simulink model "FINAL"  (R2019a)
settings: Solver=VariableStepAuto  StartTime=0.0  StopTime=5  FixedStep=0.0001  RelTol=1e-3
PreLoadFcn:
  | initDuckWPT
InitFcn:
  | initDuckWPT
StartFcn:
  | initDuckWPT
values from neighbouring files (symbols this model uses):
  angleTolerance = 2    [initDuckWPT.m]
  eeTolerance = 0.01    [initDuckWPT.m]
  JointBounds1 = [-pi/2       pi ... (first row only)    [initDuckWPT.m]
  JointBounds2 = [-pi/3       pi/3 ... (first row only)    [initDuckWPT.m]
  rotM1 = roty(90)*rotx(90)    [initDuckWPT.m]
  trajectory = [0.4  0.4  0.4  0.4  0.4  0.4  0.4 ... (first row only)    [initDuckWPT.m]
undefined symbols (not defined in the file or in its folder): DiscIntNeverNeededParam, X, Y, Z
libraries: sm_lib x205, fl_lib x72, nesl_utility x43, fl_ps_legacy_lib x18, fuzblock x16, Contact_Forces_Lib x12
(part 1 of 7)
Description:
  | Two 7-DOF Robot Arm
  | Follow Trajectory Seperate 2 Arm, No Torque, No Grabbing
settings Model: PauseTimes=4  Creator=josea  LastModifiedBy=Duke Nguyen
settings DataIOCC: ReturnWorkspaceOutputs=off
settings DebuggingCC: PregeneratedLibrarySubsystemCodeDiagnostic=none  ArithmeticOperatorsInVariantConditions=warning
settings SFSimCC: SimUseLocalCustomCode=off
settings RTWCC: RTWUseLocalCustomCode=off
settings SimscapeCC: SimscapeLogType=all  SimscapeLogName=simlog_waypoint_tracking  SimscapeLogLimitData=off
settings ExplorerConfigSet: InternalSimMechanicsExplorerSettings="<ExplorerConfiguration><canonicalview>default</canonicalview><AnimationSetting><BasePlaybackSpeed>1.0</BasePlaybackSpeed><PlaybackSpeedFactor>1.0</PlaybackSpeedFactor></AnimationSetting><TilePanel><TileInfo><Tiles Columns=\"2\" Count=\"3\" Rows=\"2\"><Column Weight=\"0.523\"/><Column Weight=\"0.477\"/><Row Weight=\"0.4994\"/><Row Weight=\"0.5006\"/><Tile Height=\"2\" Width=\"1\" X=\"0\" Y=\"0\"/><Tile Height=\"1\" Width=\"1\" X=\"1\" Y=\"0\"/><Tile Height=\"1\" Width=\"1\" X=\"1\" Y=\"1\"/></Tiles></TileInfo><SceneInfo><SceneViewer><BGColor><R>0.800000011920928955</R><G>0.800000011920928955</G><B>0.800000011920928955</B></BGColor><Camera><DoPerspective>off</DoPerspective><Position><X>1.19928295196616075</X><Y>-0.370963369649593755</Y><Z>0.192902442559522713</Z></Position><Center><X>0.466827313465554616</X><Y>0.0298302780043228633</Y><Z>-0.357436716168019419</Z></Center><Up><X>-0.458278077763030423</X><Y>0.307545069196018872</Y><Z>0.833904811027636583</Z></Up><ViewLimDist>1</ViewLimDist><YLim>0.756041493589077906</YLim><XLim>0.742600755925272082</XLim></Camera></SceneViewer><SceneViewer><BGColor><R>0.800000011920928955</R><G>0.800000011920928955</G><B>0.800000011920928955</B></BGColor><Camera><DoPerspective>off</DoPerspective><Position><X>1.51688776390650482</X><Y>-1.12635047955222944e-08</Y><Z>-0.248862136929848043</Z></Position><Center><X>0.453640252731354554</X><Y>-1.12635047955222944e-08</Y><Z>-0.248862136929848043</Z></Center><Up><X>-0</X><Y>0</Y><Z>1</Z></Up><ViewLimDist>1</ViewLimDist><YLim>0.361672012805938747</YLim><XLim>0.655073353531655411</XLim></Camera></SceneViewer><SceneViewer><BGColor><R>0.800000011920928955</R><G>0.800000011920928955</G><B>0.800000011920928955</B></BGColor><Camera><DoPerspective>off</DoPerspective><Position><X>0.45769736697222041</X><Y>-1.00000001614500644</Y><Z>-0.253455854452269813</Z></Position><Center><X>0.45769736697222041</X><Y>-1.61450063873580518e-08</Y><Z>-0.253455854452269813</Z></Center><Up><X>0</X><Y>-0</Y><Z>1</Z></Up><ViewLimDist>1</ViewLimDist><YLim>0.356940470933914178</YLim><XLim>0.645053855544248544</XLim></Camera></SceneViewer></SceneInfo></TilePanel><MechEditorPanel><Cameras/><GfxPanelCameraMap/><VideoCreator><PlaybackSpeedRatio>1.0</PlaybackSpeedRatio><FrameRate>30</FrameRate><VideoFormat>Motion JPEG AVI</VideoFormat><FrameSize>auto</FrameSize></VideoCreator></MechEditorPanel></ExplorerConfiguration>"

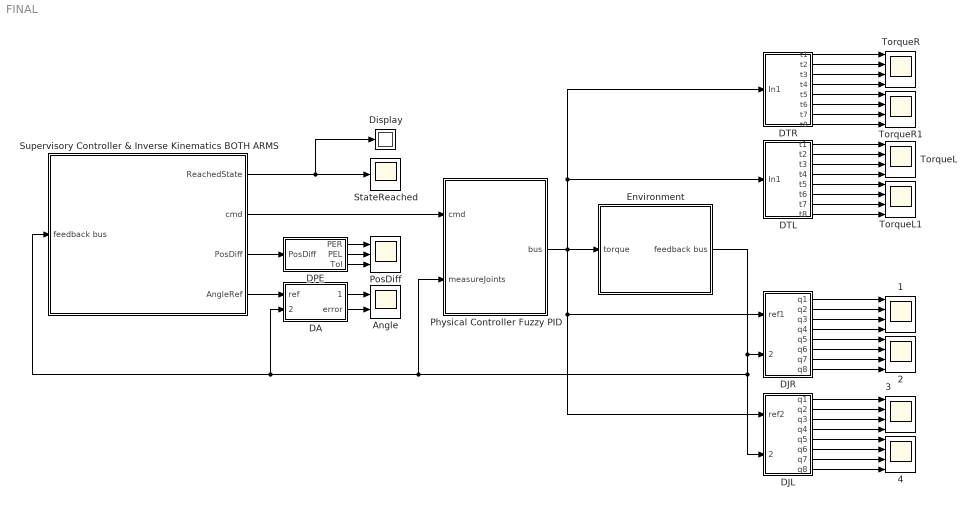
== system FINAL ==
  {1..4} (4 alike) : Scope  NumInputPorts=4
  Angle : Scope  NumInputPorts=2
  DA : Subsystem
  DJL : Subsystem
  DJR : Subsystem
  DPE : Subsystem
  DTL : Subsystem
  DTR : Subsystem
  Display : Display
  Environment : Subsystem
      mask Display: image('envi.png');
  Physical Controller Fuzzy PID : Subsystem
  PosDiff : Scope  NumInputPorts=3
  StateReached : Scope
  Supervisory Controller & Inverse Kinematics BOTH ARMS : Subsystem
  TorqueL : Scope  NumInputPorts=4
  TorqueL1 : Scope  NumInputPorts=4
  TorqueR : Scope  NumInputPorts=4
  TorqueR1 : Scope  NumInputPorts=4
  wires:
  Environment/1(feedback bus) -> Physical Controller Fuzzy PID/2(measureJoints), Supervisory Controller & Inverse Kinematics BOTH ARMS/1(feedback bus), DA/2(angle), DJL/2(meas), DJR/2(meas)
  Physical Controller Fuzzy PID/1(bus) -> DJL/1(ref2), DJR/1(ref1), Environment/1(torque), DTR/1(In1), DTL/1(In1)
  DA/1(tracking) -> Angle/1
  DA/2(error) -> Angle/2
  Supervisory Controller & Inverse Kinematics BOTH ARMS/1(ReachedState) -> Display/1, StateReached/1
  Supervisory Controller & Inverse Kinematics BOTH ARMS/3(PosDiff) -> DPE/1(PosDiff)
  DPE/1(PER) -> PosDiff/1
  DPE/2(PEL) -> PosDiff/2
  DPE/3(Tol) -> PosDiff/3
  Supervisory Controller & Inverse Kinematics BOTH ARMS/2(cmd) -> Physical Controller Fuzzy PID/1(cmd)
  Supervisory Controller & Inverse Kinematics BOTH ARMS/4(AngleRef) -> DA/1(ref)
  DTR/1(t1) -> TorqueR/1
  DTR/2(t2) -> TorqueR/2
  DTR/3(t3) -> TorqueR/3
  DTR/4(t4) -> TorqueR/4
  DTR/5(t5) -> TorqueR1/1
  DTR/6(t6) -> TorqueR1/2
  DTR/7(t7) -> TorqueR1/3
  DTR/8(t8) -> TorqueR1/4
  DTL/1(t1) -> TorqueL/1
  DTL/2(t2) -> TorqueL/2
  DTL/3(t3) -> TorqueL/3
  DTL/4(t4) -> TorqueL/4
  DTL/5(t5) -> TorqueL1/1
  DTL/6(t6) -> TorqueL1/2
  DTL/7(t7) -> TorqueL1/3
  DTL/8(t8) -> TorqueL1/4
  DJR/1(q1) -> 1/1
  DJR/2(q2) -> 1/2
  DJR/3(q3) -> 1/3
  DJR/4(q4) -> 1/4
  DJR/5(q5) -> 2/1
  DJR/6(q6) -> 2/2
  DJR/7(q7) -> 2/3
  DJR/8(q8) -> 2/4
  DJL/1(q1) -> 3/1
  DJL/2(q2) -> 3/2
  DJL/3(q3) -> 3/3
  DJL/4(q4) -> 3/4
  DJL/5(q5) -> 4/1
  DJL/6(q6) -> 4/2
  DJL/7(q7) -> 4/3
  DJL/8(q8) -> 4/4

== system FINAL/DA ==
  ref : Inport
  angle : Inport  Port=2
  Abs : Abs
  Bus Selector2 : BusSelector  OutputSignals=ObjectAngle
  Constant : Constant  Value=angleTolerance
  Mux : Mux  Inputs=2
  Mux1 : Mux  Inputs=2
  Subtract : Sum  Inputs=+-
  tracking : Outport
  error : Outport  Port=2
  wires:
  ref/1 -> Subtract/1, Mux/1
  Mux/1 -> tracking/1
  angle/1 -> Bus Selector2/1
  Bus Selector2/1 -> Subtract/2, Mux/2  "<ObjectAngle>"
  Subtract/1 -> Abs/1
  Constant/1 -> Mux1/2
  Mux1/1 -> error/1
  Abs/1 -> Mux1/1

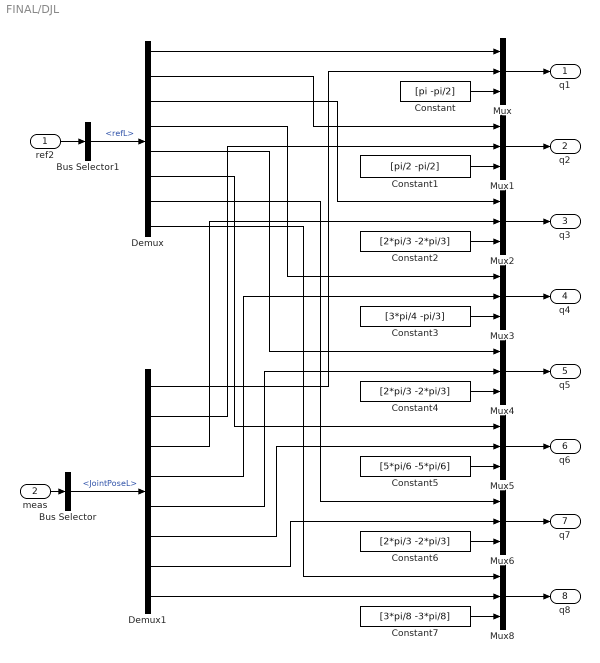
== system FINAL/DJL ==
  ref2 : Inport
  meas : Inport  Port=2
  Bus Selector : BusSelector  OutputSignals=JointPoseL
  Bus Selector1 : BusSelector  OutputSignals=refL
  Constant : Constant  Value=[pi -pi/2]
  Constant1 : Constant  Value=[pi/2 -pi/2]
  Constant2 : Constant  Value=[2*pi/3 -2*pi/3]
  Constant3 : Constant  Value=[3*pi/4 -pi/3]
  Constant4 : Constant  Value=[2*pi/3 -2*pi/3]
  Constant5 : Constant  Value=[5*pi/6 -5*pi/6]
  Constant6 : Constant  Value=[2*pi/3 -2*pi/3]
  Constant7 : Constant  Value=[3*pi/8 -3*pi/8]
  Demux : Demux  Outputs=8
  Demux1 : Demux  Outputs=8
  Mux{,1..6,8} (8 alike) : Mux  Inputs=3
  q1 : Outport
  q2 : Outport  Port=2
  q3 : Outport  Port=3
  q4 : Outport  Port=4
  q5 : Outport  Port=5
  q6 : Outport  Port=6
  q7 : Outport  Port=7
  q8 : Outport  Port=8
  wires:
  Bus Selector/1 -> Demux1/1  "<JointPoseL>"
  meas/1 -> Bus Selector/1
  Constant7/1 -> Mux8/3
  Demux/1 -> Mux/1
  Demux/2 -> Mux1/1
  Demux/3 -> Mux2/1
  Demux/4 -> Mux3/1
  Demux/5 -> Mux4/1
  Demux/6 -> Mux5/1
  Demux/7 -> Mux6/1
  Demux/8 -> Mux8/1
  Demux1/1 -> Mux/2
  Demux1/2 -> Mux1/2
  Demux1/3 -> Mux2/2
  Demux1/4 -> Mux3/2
  Demux1/5 -> Mux4/2
  Demux1/6 -> Mux5/2
  Demux1/7 -> Mux6/2
  Demux1/8 -> Mux8/2
  Constant/1 -> Mux/3
  Constant1/1 -> Mux1/3
  Constant2/1 -> Mux2/3
  Constant3/1 -> Mux3/3
  Constant4/1 -> Mux4/3
  Constant6/1 -> Mux6/3
  Constant5/1 -> Mux5/3
  Mux/1 -> q1/1
  Mux1/1 -> q2/1
  Mux2/1 -> q3/1
  Mux3/1 -> q4/1
  Mux5/1 -> q6/1
  Mux6/1 -> q7/1
  Mux8/1 -> q8/1
  Mux4/1 -> q5/1
  ref2/1 -> Bus Selector1/1
  Bus Selector1/1 -> Demux/1  "<refL>"

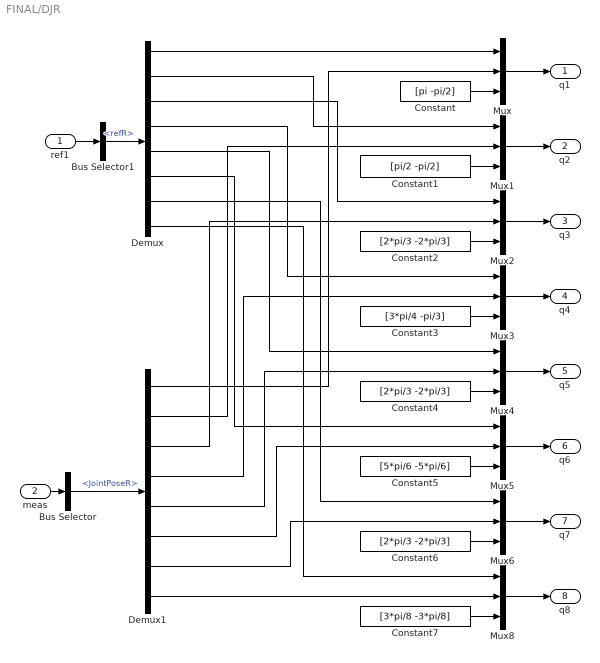
== system FINAL/DJR ==
  ref1 : Inport
  meas : Inport  Port=2
  Bus Selector : BusSelector  OutputSignals=JointPoseR
  Bus Selector1 : BusSelector  OutputSignals=refR
  Constant : Constant  Value=[pi -pi/2]
  Constant1 : Constant  Value=[pi/2 -pi/2]
  Constant2 : Constant  Value=[2*pi/3 -2*pi/3]
  Constant3 : Constant  Value=[3*pi/4 -pi/3]
  Constant4 : Constant  Value=[2*pi/3 -2*pi/3]
  Constant5 : Constant  Value=[5*pi/6 -5*pi/6]
  Constant6 : Constant  Value=[2*pi/3 -2*pi/3]
  Constant7 : Constant  Value=[3*pi/8 -3*pi/8]
  Demux : Demux  Outputs=8
  Demux1 : Demux  Outputs=8
  Mux{,1..6,8} (8 alike) : Mux  Inputs=3
  q1 : Outport
  q2 : Outport  Port=2
  q3 : Outport  Port=3
  q4 : Outport  Port=4
  q5 : Outport  Port=5
  q6 : Outport  Port=6
  q7 : Outport  Port=7
  q8 : Outport  Port=8
  wires:
  Mux4/1 -> q5/1
  Mux8/1 -> q8/1
  Mux6/1 -> q7/1
  Mux5/1 -> q6/1
  Mux3/1 -> q4/1
  Mux2/1 -> q3/1
  Mux1/1 -> q2/1
  Mux/1 -> q1/1
  Constant5/1 -> Mux5/3
  Constant6/1 -> Mux6/3
  Constant4/1 -> Mux4/3
  Constant3/1 -> Mux3/3
  Constant2/1 -> Mux2/3
  Constant1/1 -> Mux1/3
  Constant/1 -> Mux/3
  Demux1/8 -> Mux8/2
  Demux1/7 -> Mux6/2
  Demux1/6 -> Mux5/2
  Demux1/5 -> Mux4/2
  Demux1/4 -> Mux3/2
  Demux1/3 -> Mux2/2
  Demux1/2 -> Mux1/2
  Demux1/1 -> Mux/2
  Demux/8 -> Mux8/1
  Demux/7 -> Mux6/1
  Demux/6 -> Mux5/1
  Demux/5 -> Mux4/1
  Demux/4 -> Mux3/1
  Demux/3 -> Mux2/1
  Demux/2 -> Mux1/1
  Demux/1 -> Mux/1
  Constant7/1 -> Mux8/3
  meas/1 -> Bus Selector/1
  Bus Selector/1 -> Demux1/1  "<JointPoseR>"
  ref1/1 -> Bus Selector1/1
  Bus Selector1/1 -> Demux/1  "<refR>"

== system FINAL/DPE ==
  PosDiff : Inport
  Bus Selector : BusSelector  OutputSignals=PosDiffR,PosDiffL
  Constant6 : Constant  Value=eeTolerance
  Vector Length1 : Subsystem
  Vector Length2 : Subsystem
  PER : Outport
  PEL : Outport  Port=2
  Tol : Outport  Port=3
  wires:
  Bus Selector/1 -> Vector Length1/1(v)  "<PosDiffR>"
  PosDiff/1 -> Bus Selector/1
  Bus Selector/2 -> Vector Length2/1(v)  "<PosDiffL>"
  Vector Length1/1(r) -> PER/1
  Vector Length2/1(r) -> PEL/1
  Constant6/1 -> Tol/1

== system FINAL/DTL ==
  In1 : Inport
  Bus Selector3 : BusSelector  OutputSignals=torqueL
  Demux : Demux  Outputs=8
  t1 : Outport
  t2 : Outport  Port=2
  t3 : Outport  Port=3
  t4 : Outport  Port=4
  t5 : Outport  Port=5
  t6 : Outport  Port=6
  t7 : Outport  Port=7
  t8 : Outport  Port=8
  wires:
  In1/1 -> Bus Selector3/1
  Demux/4 -> t4/1
  Demux/1 -> t1/1
  Demux/7 -> t7/1
  Demux/3 -> t3/1
  Bus Selector3/1 -> Demux/1  "<torqueL>"
  Demux/2 -> t2/1
  Demux/5 -> t5/1
  Demux/8 -> t8/1
  Demux/6 -> t6/1

== system FINAL/DTR ==
  In1 : Inport
  Bus Selector2 : BusSelector  OutputSignals=torqueR
  Demux : Demux  Outputs=8
  t1 : Outport
  t2 : Outport  Port=2
  t3 : Outport  Port=3
  t4 : Outport  Port=4
  t5 : Outport  Port=5
  t6 : Outport  Port=6
  t7 : Outport  Port=7
  t8 : Outport  Port=8
  wires:
  Demux/6 -> t6/1
  Demux/4 -> t4/1
  Demux/2 -> t2/1
  Demux/5 -> t5/1
  In1/1 -> Bus Selector2/1
  Demux/7 -> t7/1
  Bus Selector2/1 -> Demux/1  "<torqueR>"
  Demux/3 -> t3/1
  Demux/8 -> t8/1
  Demux/1 -> t1/1

== system FINAL/Environment ==
  torque : Inport
  " " : Subsystem
  Bus Creator : BusCreator  Inputs=8
  Bus Selector : BusSelector  OutputSignals=torqueR,torqueL
  EE Position to World Base : Subsystem
  Rate Transition{,2,4..5} (4 alike) : RateTransition
  Robot : Subsystem  mask{damping_coefficient=2, damping_coefficient_gripper=0.14}
      mask prompts: damping_coefficient "Damping Coefficient"; damping_coefficient_gripper "Damping Coefficient Gripper"
  World : Subsystem  mask{ball_radius=3.5, contact_gripper_planeLength_x=0.05, contact_gripper_planeLength_y=0.7, contact_gripper_planeDepth=0.05, contact_gripper_stiffness=1000, contact_gripper_damping=70, contact_gripper_kFrictionCoeff=0.5, contact_gripper_sFrictionCoeff=0.72}
      mask prompts: ball_radius "Ball Radius"; contact_gripper_planeLength_x "Contact Gripper Plane Length X"; contact_gripper_planeLength_y "Contact Gripper Plane Length Y"; contact_gripper_planeDepth "Contact Gripper Plane Depth"; contact_gripper_stiffness "Contact Gripper Stiffness"; contact_gripper_damping "Contact Gripper Damping"; contact_gripper_kFrictionCoeff "Contact Gripper Kinematic Friction"; contact_gripper_sFrictionCoeff "Contact Gripper Static Friction"
  trajectoryL : ToWorkspace  VariableName=simout1  SaveFormat=Timeseries  SampleTime=-1
  trajectoryR : ToWorkspace  VariableName=simout  SaveFormat=Timeseries  SampleTime=-1
  feedback bus : Outport
  wires:
  Rate Transition/1 -> Bus Creator/1  "JointPoseR"
  Rate Transition2/1 -> Bus Creator/2  "JointPoseL"
  EE Position to World Base/1(EE1 Pos) -> Rate Transition4/1
  EE Position to World Base/2(EE2 Pos) -> Rate Transition5/1
  Rate Transition4/1 -> Bus Creator/3, trajectoryR/1  "EERPos"
  Rate Transition5/1 -> trajectoryL/1, Bus Creator/4  "EELPose"
  Robot/1(SensorData1) -> Rate Transition/1
  Robot/2(SensorData2) -> Rate Transition2/1
  World/1(ObjectPosition) -> Bus Creator/5  "Object Position"
  World/3(GripperForce2) -> Bus Creator/7  "GripForceL"
  World/2(GripperForce1) -> Bus Creator/6  "GripForceR"
  Bus Creator/1 -> feedback bus/1
  World/4(ObjectAngle) -> Bus Creator/8  "ObjectAngle"
  torque/1 -> Bus Selector/1
  Bus Selector/1 -> Robot/1(commandsRight)  "<torqueR>"
  Bus Selector/2 -> Robot/2(commandsLeft)  "<torqueL>"
  connections:
  Robot/LConn2 -- EE Position to World Base/LConn1
  Robot/LConn3 -- EE Position to World Base/LConn2
  " "/RConn1 -- World/LConn1 -- EE Position to World Base/LConn3 -- Robot/LConn1
  Robot/RConn1 -- World/RConn1
  Robot/RConn2 -- World/RConn3
  Robot/RConn3 -- World/RConn2
  World/RConn4 -- Robot/RConn4

== system FINAL/Physical Controller Fuzzy PID ==
  cmd : Inport
  measureJoints : Inport  Port=2
  Bus Creator : BusCreator  Inputs=4
  Bus Selector : BusSelector  OutputSignals=JointPoseR,JointPoseL
  Bus Selector1 : BusSelector  OutputSignals=DesiredJointStatesR,GripCommand,DesiredJointStatesL
  Fuzzy PID Tuning1 : Subsystem
  Fuzzy PID Tuning2 : Subsystem
  Grip Transition : Subsystem
  Mux1 : Mux  Inputs=2
  Mux2 : Mux  Inputs=2
  bus : Outport
  wires:
  Fuzzy PID Tuning1/1(Out1) -> Bus Creator/2  "torqueR"
  Fuzzy PID Tuning2/1(Out1) -> Bus Creator/3  "torqueL"
  Bus Selector1/2 -> Grip Transition/1(GripCmd)  "<GripCommand>"
  Bus Selector1/3 -> Mux1/1  "<DesiredJointStatesL>"
  Bus Selector/2 -> Fuzzy PID Tuning2/2(In2)  "<JointPoseL>"
  Grip Transition/1(GripRef) -> Mux2/2, Mux1/2
  Mux2/1 -> Fuzzy PID Tuning1/1(In1), Bus Creator/1  "refR"
  Bus Selector1/1 -> Mux2/1  "<DesiredJointStatesR>"
  Bus Creator/1 -> bus/1
  Bus Selector/1 -> Fuzzy PID Tuning1/2(In2)  "<JointPoseR>"
  Mux1/1 -> Fuzzy PID Tuning2/1(In1), Bus Creator/4  "refL"
  cmd/1 -> Bus Selector1/1
  measureJoints/1 -> Bus Selector/1

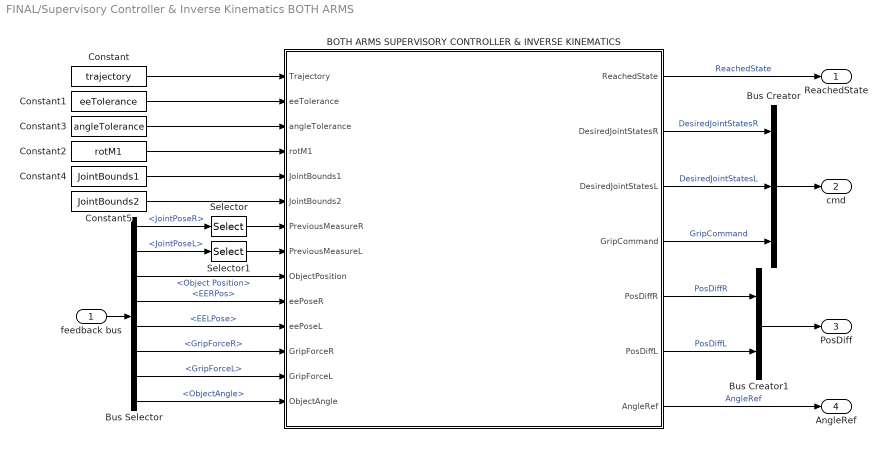
== system FINAL/Supervisory Controller & Inverse Kinematics BOTH ARMS ==
  feedback bus : Inport
  BOTH ARMS SUPERVISORY CONTROLLER & INVERSE KINEMATICS : Stateflow chart  TreatAsAtomicUnit=on
  Bus Creator : BusCreator  Inputs=3
  Bus Creator1 : BusCreator  Inputs=2
  Bus Selector : BusSelector  OutputSignals=JointPoseR,JointPoseL,Object Position,EERPos,EELPose,GripForceR,GripForceL,ObjectAngle
  Constant : Constant  Value=trajectory
  Constant1 : Constant  Value=eeTolerance
  Constant2 : Constant  Value=rotM1
  Constant3 : Constant  Value=angleTolerance
  Constant4 : Constant  Value=JointBounds1
  Constant5 : Constant  Value=JointBounds2
  Selector : Selector  InputPortWidth=8  IndexOptions=Index vector (dialog)  Indices=[1:7]  OutputSizes=1
  Selector1 : Selector  InputPortWidth=8  IndexOptions=Index vector (dialog)  Indices=[1:7]  OutputSizes=1
  ReachedState : Outport
  cmd : Outport  Port=2
  PosDiff : Outport  Port=3
  AngleRef : Outport  Port=4
  wires:
  Selector/1 -> BOTH ARMS SUPERVISORY CONTROLLER & INVERSE KINEMATICS/7(PreviousMeasureR)
  Constant2/1 -> BOTH ARMS SUPERVISORY CONTROLLER & INVERSE KINEMATICS/4(rotM1)
  Bus Selector/6 -> BOTH ARMS SUPERVISORY CONTROLLER & INVERSE KINEMATICS/12(GripForceR)  "<GripForceR>"
  Constant5/1 -> BOTH ARMS SUPERVISORY CONTROLLER & INVERSE KINEMATICS/6(JointBounds2)
  feedback bus/1 -> Bus Selector/1
  Constant1/1 -> BOTH ARMS SUPERVISORY CONTROLLER & INVERSE KINEMATICS/2(eeTolerance)
  Constant/1 -> BOTH ARMS SUPERVISORY CONTROLLER & INVERSE KINEMATICS/1(Trajectory)
  Constant4/1 -> BOTH ARMS SUPERVISORY CONTROLLER & INVERSE KINEMATICS/5(JointBounds1)
  Selector1/1 -> BOTH ARMS SUPERVISORY CONTROLLER & INVERSE KINEMATICS/8(PreviousMeasureL)
  Bus Selector/2 -> Selector1/1  "<JointPoseL>"
  Bus Selector/7 -> BOTH ARMS SUPERVISORY CONTROLLER & INVERSE KINEMATICS/13(GripForceL)  "<GripForceL>"
  Bus Selector/5 -> BOTH ARMS SUPERVISORY CONTROLLER & INVERSE KINEMATICS/11(eePoseL)  "<EELPose>"
  Bus Selector/1 -> Selector/1  "<JointPoseR>"
  Bus Selector/3 -> BOTH ARMS SUPERVISORY CONTROLLER & INVERSE KINEMATICS/9(ObjectPosition)  "<Object Position>"
  Bus Selector/8 -> BOTH ARMS SUPERVISORY CONTROLLER & INVERSE KINEMATICS/14(ObjectAngle)  "<ObjectAngle>"
  Bus Selector/4 -> BOTH ARMS SUPERVISORY CONTROLLER & INVERSE KINEMATICS/10(eePoseR)  "<EERPos>"
  BOTH ARMS SUPERVISORY CONTROLLER & INVERSE KINEMATICS/2(DesiredJointStatesR) -> Bus Creator/1  "DesiredJointStatesR"
  BOTH ARMS SUPERVISORY CONTROLLER & INVERSE KINEMATICS/3(DesiredJointStatesL) -> Bus Creator/2  "DesiredJointStatesL"
  BOTH ARMS SUPERVISORY CONTROLLER & INVERSE KINEMATICS/4(GripCommand) -> Bus Creator/3  "GripCommand"
  BOTH ARMS SUPERVISORY CONTROLLER & INVERSE KINEMATICS/1(ReachedState) -> ReachedState/1  "ReachedState"
  Bus Creator/1 -> cmd/1
  BOTH ARMS SUPERVISORY CONTROLLER & INVERSE KINEMATICS/5(PosDiffR) -> Bus Creator1/1  "PosDiffR"
  BOTH ARMS SUPERVISORY CONTROLLER & INVERSE KINEMATICS/6(PosDiffL) -> Bus Creator1/2  "PosDiffL"
  Bus Creator1/1 -> PosDiff/1
  BOTH ARMS SUPERVISORY CONTROLLER & INVERSE KINEMATICS/7(AngleRef) -> AngleRef/1  "AngleRef"
  Constant3/1 -> BOTH ARMS SUPERVISORY CONTROLLER & INVERSE KINEMATICS/3(angleTolerance)

== system FINAL/DPE/Vector Length1 ==
  v : Inport
  Demux : Demux  Outputs=3
  Sqrt : Sqrt  SaturateOnIntegerOverflow=on
  Square : Math  Operator=square  SaturateOnIntegerOverflow=on
  Square1 : Math  Operator=square  SaturateOnIntegerOverflow=on
  Square2 : Math  Operator=square  SaturateOnIntegerOverflow=on
  Sum : Sum  Inputs=+++
  r : Outport
  wires:
  Square1/1 -> Sum/2
  Sqrt/1 -> r/1
  Demux/3 -> Square2/1
  Sum/1 -> Sqrt/1
  v/1 -> Demux/1
  Demux/2 -> Square1/1
  Demux/1 -> Square/1
  Square2/1 -> Sum/3
  Square/1 -> Sum/1

== system FINAL/DPE/Vector Length2 ==
  v : Inport
  Demux : Demux  Outputs=3
  Sqrt : Sqrt  SaturateOnIntegerOverflow=on
  Square : Math  Operator=square  SaturateOnIntegerOverflow=on
  Square1 : Math  Operator=square  SaturateOnIntegerOverflow=on
  Square2 : Math  Operator=square  SaturateOnIntegerOverflow=on
  Sum : Sum  Inputs=+++
  r : Outport
  wires:
  Square/1 -> Sum/1
  Square2/1 -> Sum/3
  Demux/1 -> Square/1
  Demux/2 -> Square1/1
  v/1 -> Demux/1
  Sum/1 -> Sqrt/1
  Demux/3 -> Square2/1
  Sqrt/1 -> r/1
  Square1/1 -> Sum/2

== system FINAL/Environment/  ==
  MechanismConfiguration : sm_lib/Utilities/Mechanism Configuration  UniformGravity=Constant  GravityVector=[0 0 -9.80665]  GravityUnits=m/s^2  LinearizationDelta=0.001
  Solver Configuration : nesl_utility/Solver Configuration  PhysicalDomain=network_engine_domain  SubClassName=solver  LeftPortType=input  RightPortType=generic  Tones=[]  Harmonics=[]  SimulateNoise=off  Profile=off  UseLocalSampling=off  EnableSwitchedLinearOptims=on  FrequencyDomain=off  UseCCode=off  RelTol=0.001  AbsTol=1e-06  MinStep=1e-09  ToWorkspace=off  RevertToSquareIcSolve=off  NumHomotopyIterations=100  PhasorMode=off  PhasorModeNumHarmonics=1  DoDC=off  ResidualTolerance=1e-09  UseLocalSolver=off  LocalSolverChoice=NE_BACKWARD_EULER_ADVANCER  LocalSolverSampleTime=0.001  DoFixedCost=off  MaxNonlinIter=3  MaxModeIter=2  LinearAlgebra=Sparse  EquationFormulation=NE_TIME_EF  DelaysMemoryBudget=1024  AutomaticFiltering=on  FilteringTimeConstant=0.001  PartitionStorageMethod=AS_NEEDED  PartitionMemoryBudget=1024  PartitionMethod=FAST
  World1 : sm_lib/Frames and Transforms/World Frame
  WC : PMIOPort  Side=Right
  connections:
  World1/RConn1 -- WC/RConn1 -- Solver Configuration/RConn1 -- MechanismConfiguration/RConn1

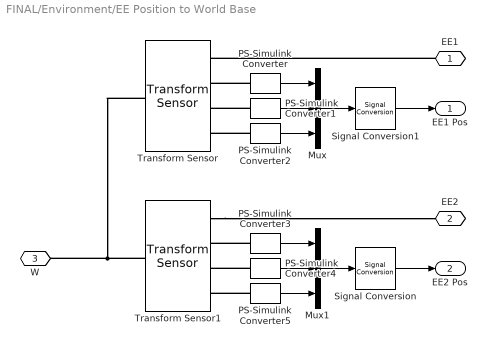
== system FINAL/Environment/EE Position to World Base ==
  Mux : Mux  Inputs=3
  Mux1 : Mux  Inputs=3
  PS-Simulink Converter{,1..5} (6 alike) : nesl_utility/PS-Simulink Converter  PhysicalDomain=network_engine_domain  SubClassName=ps_output  LeftPortType=input  RightPortType=output  PseudoPeriodic=off  Frequencies=[]  Unit=1  AffineConversion=off
  Signal Conversion : SignalConversion  OverrideOpt=off
  Signal Conversion1 : SignalConversion  OverrideOpt=off
  Transform Sensor : sm_lib/Frames and Transforms/Transform Sensor  MeasurementFrame=World  SenseAngle=off  SenseAxis=off  SenseAngle1=off  SenseAngle2=off  SenseAngle3=off  SenseQ=off  SenseR=off  SenseOmegaX=off  SenseOmegaY=off  SenseOmegaZ=off  SenseOmega1=off  SenseOmega2=off  SenseOmega3=off  SenseQDot=off  SenseRDot=off  SenseAlphaX=off  SenseAlphaY=off  SenseAlphaZ=off  SenseAlpha1=off  SenseAlpha2=off  SenseAlpha3=off  SenseQDDot=off  SenseRDDot=off  SenseX=on  SenseY=on  SenseZ=on  SenseRad=off  SenseAzim=off  SenseDist=off  SenseInc=off  SenseXDot=off  SenseYDot=off  SenseZDot=off  SenseRadDot=off  SenseAzimDot=off  SenseDistDot=off  SenseIncDot=off  SenseXDDot=off  SenseYDDot=off  SenseZDDot=off  SenseRadDDot=off  SenseAzimDDot=off  SenseDistDDot=off  SenseIncDDot=off
  Transform Sensor1 : sm_lib/Frames and Transforms/Transform Sensor  MeasurementFrame=World  SenseAngle=off  SenseAxis=off  SenseAngle1=off  SenseAngle2=off  SenseAngle3=off  SenseQ=off  SenseR=off  SenseOmegaX=off  SenseOmegaY=off  SenseOmegaZ=off  SenseOmega1=off  SenseOmega2=off  SenseOmega3=off  SenseQDot=off  SenseRDot=off  SenseAlphaX=off  SenseAlphaY=off  SenseAlphaZ=off  SenseAlpha1=off  SenseAlpha2=off  SenseAlpha3=off  SenseQDDot=off  SenseRDDot=off  SenseX=on  SenseY=on  SenseZ=on  SenseRad=off  SenseAzim=off  SenseDist=off  SenseInc=off  SenseXDot=off  SenseYDot=off  SenseZDot=off  SenseRadDot=off  SenseAzimDot=off  SenseDistDot=off  SenseIncDot=off  SenseXDDot=off  SenseYDDot=off  SenseZDDot=off  SenseRadDDot=off  SenseAzimDDot=off  SenseDistDDot=off  SenseIncDDot=off
  EE1 : PMIOPort  Side=Left
  EE2 : PMIOPort  Port=2  Side=Left
  W : PMIOPort  Port=3  Side=Left
  EE1 Pos : Outport
  EE2 Pos : Outport  Port=2
  wires:
  PS-Simulink Converter1/1 -> Mux/2
  PS-Simulink Converter3/1 -> Mux1/1
  PS-Simulink Converter/1 -> Mux/1
  PS-Simulink Converter2/1 -> Mux/3
  PS-Simulink Converter4/1 -> Mux1/2
  PS-Simulink Converter5/1 -> Mux1/3
  Mux/1 -> Signal Conversion1/1
  Mux1/1 -> Signal Conversion/1
  Signal Conversion/1 -> EE2 Pos/1
  Signal Conversion1/1 -> EE1 Pos/1
  connections:
  PS-Simulink Converter5/LConn1 -- Transform Sensor1/RConn4
  PS-Simulink Converter3/LConn1 -- Transform Sensor1/RConn2
  Transform Sensor1/LConn1 -- Transform Sensor/LConn1 -- W/RConn1
  EE1/RConn1 -- Transform Sensor/RConn1
  PS-Simulink Converter4/LConn1 -- Transform Sensor1/RConn3
  PS-Simulink Converter/LConn1 -- Transform Sensor/RConn2
  PS-Simulink Converter1/LConn1 -- Transform Sensor/RConn3
  PS-Simulink Converter2/LConn1 -- Transform Sensor/RConn4
  Transform Sensor1/RConn1 -- EE2/RConn1
